simulink model "LUT_kidney_25"  (R2023b)
settings: Solver=FixedStepAuto  StartTime=0  StopTime=10.1  FixedStep=Timegap  RelTol=1e-3
model workspace (MAT data in the model file):
  T1_input = 1.34
(part 1 of 3)
settings Model: Creator=ppxmr2  LastModifiedBy=ppxmr2

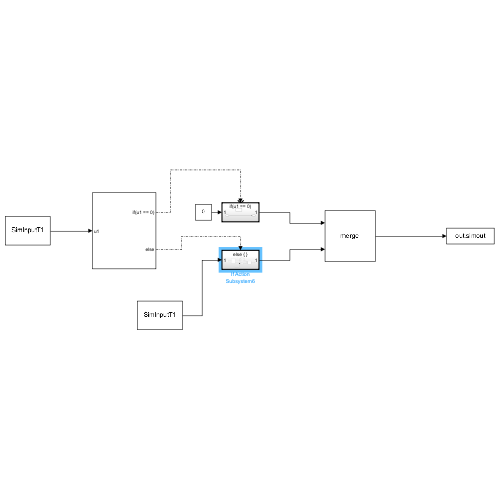
[thumbnail: Simulink's stored preview of the top-level diagram]
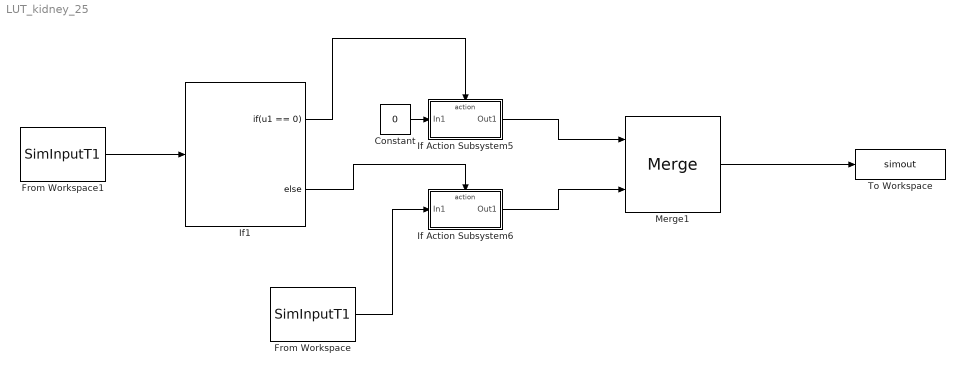
== system LUT_kidney_25 ==
  Constant : Constant  Value=0
  From Workspace : FromWorkspace  VariableName=SimInputT1  Interpolate=off  OutputAfterFinalValue=Setting to zero
  From Workspace1 : FromWorkspace  VariableName=SimInputT1  Interpolate=off  OutputAfterFinalValue=Setting to zero
  If Action Subsystem5 : Subsystem  TreatAsAtomicUnit=on
  If Action Subsystem6 : Subsystem  TreatAsAtomicUnit=on
  If1 : If  IfExpression=u1 == 0
  Merge1 : Merge
  To Workspace : ToWorkspace  VariableName=simout
  wires:
  From Workspace1/1 -> If1/1
  If1/1 -> If Action Subsystem5/Action
  If1/2 -> If Action Subsystem6/Action
  Constant/1 -> If Action Subsystem5/1(In1)
  If Action Subsystem5/1(Out1) -> Merge1/1
  If Action Subsystem6/1(Out1) -> Merge1/2
  Merge1/1 -> To Workspace/1
  From Workspace/1 -> If Action Subsystem6/1(In1)

== system LUT_kidney_25/If Action Subsystem5 ==
  In1 : Inport
  Action Port : ActionPort  ActionPortLabel=if(u1 == 0)
  Out1 : Outport
  wires:
  In1/1 -> Out1/1

== system LUT_kidney_25/If Action Subsystem6 ==
  In1 : Inport
  Action Port : ActionPort  ActionPortLabel=else
  From Workspace1 : FromWorkspace  VariableName=SimInputHR  Interpolate=off  OutputAfterFinalValue=Setting to zero
  If : If  IfExpression=u1 >= 1.495  ElseIfExpressions=u1 >= 0.995
  If Action Subsystem1 : Subsystem  TreatAsAtomicUnit=on
  If Action Subsystem2 : Subsystem  TreatAsAtomicUnit=on
  If Action Subsystem3 : Subsystem  TreatAsAtomicUnit=on
  Merge : Merge  Inputs=3
  Out1 : Outport
  wires:
  Merge/1 -> Out1/1
  From Workspace1/1 -> If/1
  If Action Subsystem1/1(Out1) -> Merge/2
  If Action Subsystem3/1(Out1) -> Merge/3
  In1/1 -> If Action Subsystem2/1(In1), If Action Subsystem1/1(In1), If Action Subsystem3/1(In1)
  If/1 -> If Action Subsystem2/Action
  If/2 -> If Action Subsystem1/Action
  If/3 -> If Action Subsystem3/Action
  If Action Subsystem2/1(Out1) -> Merge/1

== system LUT_kidney_25/If Action Subsystem6/If Action Subsystem1 ==
  In1 : Inport
  Action Port : ActionPort  ActionPortLabel=elseif(u1 >= 0.995)
  From Workspace2 : FromWorkspace  VariableName=SimInputHR  Interpolate=off  OutputAfterFinalValue=Setting to zero
  If Action Subsystem5 : Subsystem  TreatAsAtomicUnit=on
  If Action Subsystem6 : Subsystem  TreatAsAtomicUnit=on
  If Action Subsystem7 : Subsystem  TreatAsAtomicUnit=on
  If Action Subsystem8 : Subsystem  TreatAsAtomicUnit=on
  If Action Subsystem9 : Subsystem  TreatAsAtomicUnit=on
  If1 : If  IfExpression=u1 >= 1.395  ElseIfExpressions=u1 >= 1.295, u1 >= 1.195, u1 >= 1.095
  Merge1 : Merge  Inputs=5
  Out1 : Outport
  wires:
  In1/1 -> If Action Subsystem7/1(In2), If Action Subsystem8/1(In1), If Action Subsystem9/1(In1), If Action Subsystem5/1(In1), If Action Subsystem6/1(In1)
  From Workspace2/1 -> If1/1
  If Action Subsystem9/1(Out1) -> Merge1/1
  If Action Subsystem6/1(Out1) -> Merge1/5
  If Action Subsystem8/1(Out1) -> Merge1/2
  If Action Subsystem5/1(Out1) -> Merge1/4
  If1/4 -> If Action Subsystem5/Action
  If1/2 -> If Action Subsystem8/Action
  If1/3 -> If Action Subsystem7/Action
  If Action Subsystem7/1(Out2) -> Merge1/3
  If1/5 -> If Action Subsystem6/Action
  If1/1 -> If Action Subsystem9/Action
  Merge1/1 -> Out1/1

== system LUT_kidney_25/If Action Subsystem6/If Action Subsystem2 ==
  In1 : Inport
  Action Port : ActionPort  ActionPortLabel=if(u1 >= 1.495)
  From Workspace2 : FromWorkspace  VariableName=SimInputHR  Interpolate=off  OutputAfterFinalValue=Setting to zero
  If Action Subsystem5 : Subsystem  TreatAsAtomicUnit=on
  If Action Subsystem6 : Subsystem  TreatAsAtomicUnit=on
  If Action Subsystem7 : Subsystem  TreatAsAtomicUnit=on
  If Action Subsystem8 : Subsystem  TreatAsAtomicUnit=on
  If Action Subsystem9 : Subsystem  TreatAsAtomicUnit=on
  If1 : If  IfExpression=u1 >= 1.895  ElseIfExpressions=u1 >= 1.795, u1 >= 1.695, u1 >= 1.595
  Merge1 : Merge  Inputs=5
  Out1 : Outport
  wires:
  In1/1 -> If Action Subsystem9/1(In1), If Action Subsystem8/1(In1), If Action Subsystem7/1(In1), If Action Subsystem5/1(In1), If Action Subsystem6/1(In1)
  From Workspace2/1 -> If1/1
  If Action Subsystem9/1(Out1) -> Merge1/1
  If1/4 -> If Action Subsystem5/Action
  If1/2 -> If Action Subsystem8/Action
  If1/3 -> If Action Subsystem7/Action
  If1/5 -> If Action Subsystem6/Action
  If1/1 -> If Action Subsystem9/Action
  Merge1/1 -> Out1/1
  If Action Subsystem8/1(Out1) -> Merge1/2
  If Action Subsystem7/1(Out1) -> Merge1/3
  If Action Subsystem6/1(Out1) -> Merge1/5
  If Action Subsystem5/1(Out1) -> Merge1/4

== system LUT_kidney_25/If Action Subsystem6/If Action Subsystem3 ==
  In1 : Inport
  Action Port : ActionPort  ActionPortLabel=else
  From Workspace2 : FromWorkspace  VariableName=SimInputHR  Interpolate=off  OutputAfterFinalValue=Setting to zero
  If Action Subsystem5 : Subsystem  TreatAsAtomicUnit=on
  If Action Subsystem6 : Subsystem  TreatAsAtomicUnit=on
  If Action Subsystem7 : Subsystem  TreatAsAtomicUnit=on
  If Action Subsystem8 : Subsystem  TreatAsAtomicUnit=on
  If Action Subsystem9 : Subsystem  TreatAsAtomicUnit=on
  If1 : If  IfExpression=u1 >= 0.895  ElseIfExpressions=u1 >= 0.795, u1 >= 0.695, u1 >= 0595
  Merge1 : Merge  Inputs=5
  Out1 : Outport
  wires:
  In1/1 -> If Action Subsystem8/1(In1), If Action Subsystem9/1(In2), If Action Subsystem7/1(In1), If Action Subsystem5/1(In1), If Action Subsystem6/1(In1)
  From Workspace2/1 -> If1/1
  If Action Subsystem9/1(Out2) -> Merge1/1
  If Action Subsystem6/1(Out1) -> Merge1/5
  If Action Subsystem8/1(Out1) -> Merge1/2
  If Action Subsystem5/1(Out1) -> Merge1/4
  If1/4 -> If Action Subsystem5/Action
  If1/2 -> If Action Subsystem8/Action
  If1/3 -> If Action Subsystem7/Action
  If Action Subsystem7/1(Out1) -> Merge1/3
  If1/5 -> If Action Subsystem6/Action
  If1/1 -> If Action Subsystem9/Action
  Merge1/1 -> Out1/1

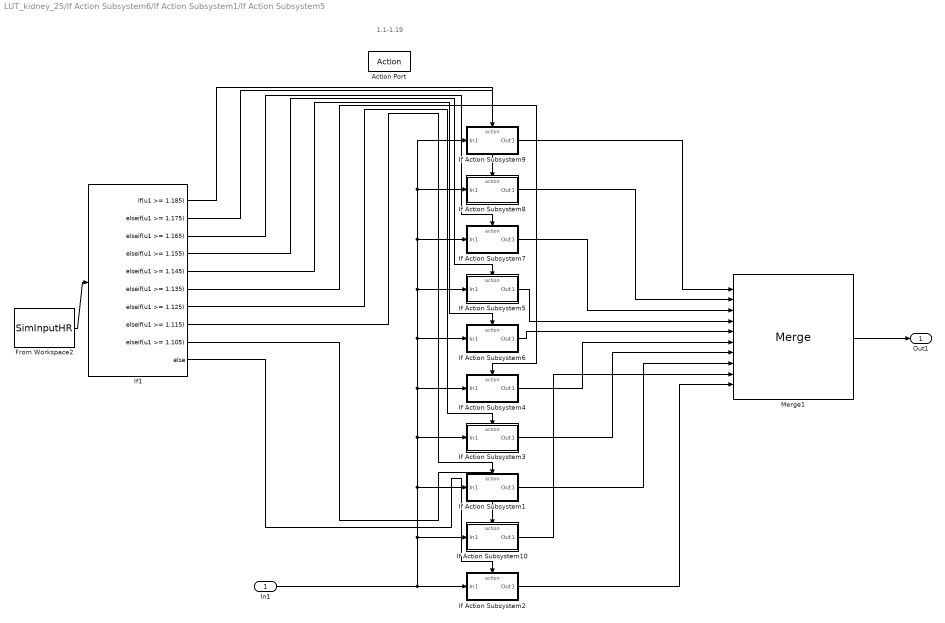
== system LUT_kidney_25/If Action Subsystem6/If Action Subsystem1/If Action Subsystem5 ==
  note: 1.1-1.19
  In1 : Inport
  Action Port : ActionPort  ActionPortLabel=elseif( u1 >= 1.095)
  From Workspace2 : FromWorkspace  VariableName=SimInputHR  Interpolate=off  OutputAfterFinalValue=Setting to zero
  If Action Subsystem1 : Subsystem  TreatAsAtomicUnit=on
  If Action Subsystem10 : Subsystem  TreatAsAtomicUnit=on
  If Action Subsystem2 : Subsystem  TreatAsAtomicUnit=on
  If Action Subsystem3 : Subsystem  TreatAsAtomicUnit=on
  If Action Subsystem4 : Subsystem  TreatAsAtomicUnit=on
  If Action Subsystem5 : Subsystem  TreatAsAtomicUnit=on
  If Action Subsystem6 : Subsystem  TreatAsAtomicUnit=on
  If Action Subsystem7 : Subsystem  TreatAsAtomicUnit=on
  If Action Subsystem8 : Subsystem  TreatAsAtomicUnit=on
  If Action Subsystem9 : Subsystem  TreatAsAtomicUnit=on
  If1 : If  IfExpression=u1 >= 1.185  ElseIfExpressions=u1 >= 1.175, u1 >= 1.165, u1 >= 1.155, u1 >= 1.145, u1 >= 1.135, u1 >= 1.125, u1 >= 1.115, u1 >= 1.105
  Merge1 : Merge  Inputs=10
  Out1 : Outport
  wires:
  If1/10 -> If Action Subsystem2/Action
  If Action Subsystem4/1(Out1) -> Merge1/6
  From Workspace2/1 -> If1/1
  If Action Subsystem6/1(Out1) -> Merge1/5
  Merge1/1 -> Out1/1
  If1/8 -> If Action Subsystem1/Action
  If Action Subsystem3/1(Out1) -> Merge1/7
  In1/1 -> If Action Subsystem1/1(In1), If Action Subsystem3/1(In1), If Action Subsystem4/1(In1), If Action Subsystem7/1(In1), If Action Subsystem8/1(In1), If Action Subsystem9/1(In1), If Action Subsystem5/1(In1), If Action Subsystem6/1(In1), If Action Subsystem10/1(In1), If Action Subsystem2/1(In1)
  If1/6 -> If Action Subsystem4/Action
  If Action Subsystem1/1(Out1) -> Merge1/8
  If1/4 -> If Action Subsystem5/Action
  If Action Subsystem8/1(Out1) -> Merge1/2
  If1/5 -> If Action Subsystem6/Action
  If Action Subsystem7/1(Out1) -> Merge1/3
  If1/3 -> If Action Subsystem7/Action
  If1/7 -> If Action Subsystem3/Action
  If Action Subsystem5/1(Out1) -> Merge1/4
  If Action Subsystem2/1(Out1) -> Merge1/10
  If1/2 -> If Action Subsystem8/Action
  If1/1 -> If Action Subsystem9/Action
  If Action Subsystem9/1(Out1) -> Merge1/1
  If1/9 -> If Action Subsystem10/Action
  If Action Subsystem10/1(Out1) -> Merge1/9

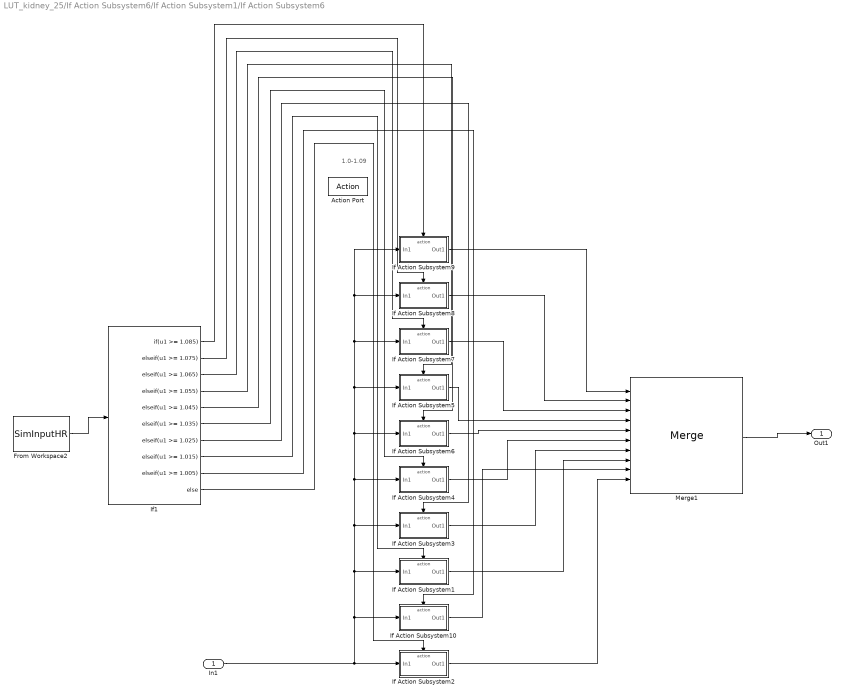
== system LUT_kidney_25/If Action Subsystem6/If Action Subsystem1/If Action Subsystem6 ==
  note: 1.0-1.09
  In1 : Inport
  Action Port : ActionPort  ActionPortLabel=else
  From Workspace2 : FromWorkspace  VariableName=SimInputHR  Interpolate=off  OutputAfterFinalValue=Setting to zero
  If Action Subsystem1 : Subsystem  TreatAsAtomicUnit=on
  If Action Subsystem10 : Subsystem  TreatAsAtomicUnit=on
  If Action Subsystem2 : Subsystem  TreatAsAtomicUnit=on
  If Action Subsystem3 : Subsystem  TreatAsAtomicUnit=on
  If Action Subsystem4 : Subsystem  TreatAsAtomicUnit=on
  If Action Subsystem5 : Subsystem  TreatAsAtomicUnit=on
  If Action Subsystem6 : Subsystem  TreatAsAtomicUnit=on
  If Action Subsystem7 : Subsystem  TreatAsAtomicUnit=on
  If Action Subsystem8 : Subsystem  TreatAsAtomicUnit=on
  If Action Subsystem9 : Subsystem  TreatAsAtomicUnit=on
  If1 : If  IfExpression=u1 >= 1.085  ElseIfExpressions=u1 >= 1.075, u1 >= 1.065, u1 >= 1.055, u1 >= 1.045, u1 >= 1.035, u1 >= 1.025, u1 >= 1.015, u1 >= 1.005
  Merge1 : Merge  Inputs=10
  Out1 : Outport
  wires:
  If1/10 -> If Action Subsystem2/Action
  If Action Subsystem4/1(Out1) -> Merge1/6
  From Workspace2/1 -> If1/1
  If Action Subsystem6/1(Out1) -> Merge1/5
  Merge1/1 -> Out1/1
  If1/8 -> If Action Subsystem1/Action
  If Action Subsystem3/1(Out1) -> Merge1/7
  In1/1 -> If Action Subsystem1/1(In1), If Action Subsystem3/1(In1), If Action Subsystem4/1(In1), If Action Subsystem7/1(In1), If Action Subsystem8/1(In1), If Action Subsystem9/1(In1), If Action Subsystem5/1(In1), If Action Subsystem6/1(In1), If Action Subsystem10/1(In1), If Action Subsystem2/1(In1)
  If1/6 -> If Action Subsystem4/Action
  If Action Subsystem1/1(Out1) -> Merge1/8
  If1/4 -> If Action Subsystem5/Action
  If Action Subsystem8/1(Out1) -> Merge1/2
  If1/5 -> If Action Subsystem6/Action
  If Action Subsystem7/1(Out1) -> Merge1/3
  If1/3 -> If Action Subsystem7/Action
  If1/7 -> If Action Subsystem3/Action
  If Action Subsystem5/1(Out1) -> Merge1/4
  If Action Subsystem2/1(Out1) -> Merge1/10
  If1/2 -> If Action Subsystem8/Action
  If1/1 -> If Action Subsystem9/Action
  If Action Subsystem9/1(Out1) -> Merge1/1
  If1/9 -> If Action Subsystem10/Action
  If Action Subsystem10/1(Out1) -> Merge1/9

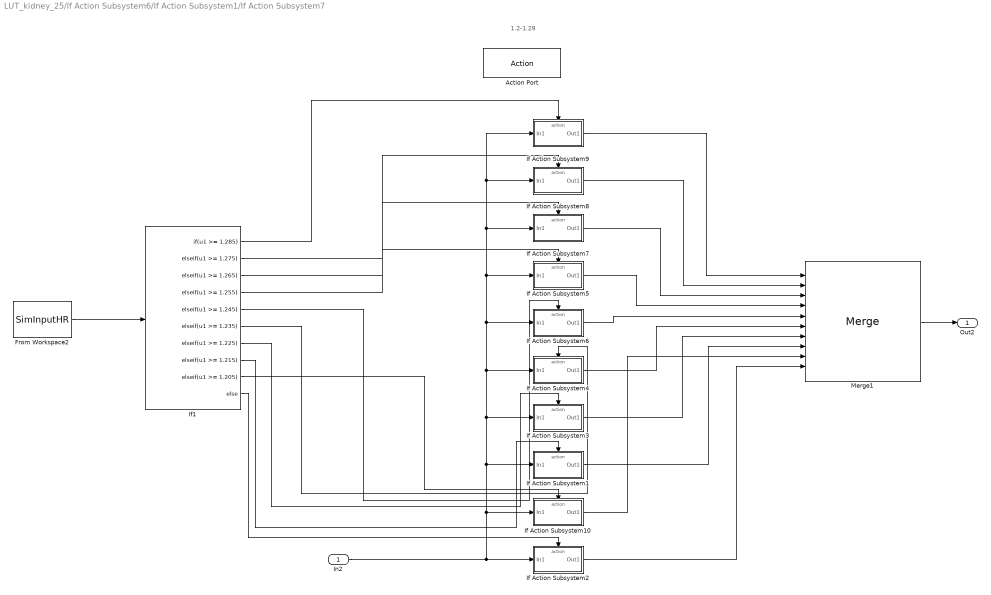
== system LUT_kidney_25/If Action Subsystem6/If Action Subsystem1/If Action Subsystem7 ==
  note: 1.2-1.29
  In2 : Inport
  Action Port : ActionPort  ActionPortLabel=elseif( u1 >= 1.195)
  From Workspace2 : FromWorkspace  VariableName=SimInputHR  Interpolate=off  OutputAfterFinalValue=Setting to zero
  If Action Subsystem1 : Subsystem  TreatAsAtomicUnit=on
  If Action Subsystem10 : Subsystem  TreatAsAtomicUnit=on
  If Action Subsystem2 : Subsystem  TreatAsAtomicUnit=on
  If Action Subsystem3 : Subsystem  TreatAsAtomicUnit=on
  If Action Subsystem4 : Subsystem  TreatAsAtomicUnit=on
  If Action Subsystem5 : Subsystem  TreatAsAtomicUnit=on
  If Action Subsystem6 : Subsystem  TreatAsAtomicUnit=on
  If Action Subsystem7 : Subsystem  TreatAsAtomicUnit=on
  If Action Subsystem8 : Subsystem  TreatAsAtomicUnit=on
  If Action Subsystem9 : Subsystem  TreatAsAtomicUnit=on
  If1 : If  IfExpression=u1 >= 1.285  ElseIfExpressions=u1 >= 1.275, u1 >= 1.265, u1 >= 1.255, u1 >= 1.245, u1 >= 1.235, u1 >= 1.225, u1 >= 1.215, u1 >= 1.205
  Merge1 : Merge  Inputs=10
  Out2 : Outport
  wires:
  If1/10 -> If Action Subsystem2/Action
  If Action Subsystem4/1(Out1) -> Merge1/6
  From Workspace2/1 -> If1/1
  If Action Subsystem6/1(Out1) -> Merge1/5
  Merge1/1 -> Out2/1
  If1/8 -> If Action Subsystem1/Action
  If Action Subsystem3/1(Out1) -> Merge1/7
  In2/1 -> If Action Subsystem1/1(In1), If Action Subsystem3/1(In1), If Action Subsystem4/1(In1), If Action Subsystem7/1(In1), If Action Subsystem8/1(In1), If Action Subsystem9/1(In1), If Action Subsystem5/1(In1), If Action Subsystem6/1(In1), If Action Subsystem10/1(In1), If Action Subsystem2/1(In1)
  If1/6 -> If Action Subsystem4/Action
  If Action Subsystem1/1(Out1) -> Merge1/8
  If1/4 -> If Action Subsystem5/Action
  If Action Subsystem8/1(Out1) -> Merge1/2
  If1/5 -> If Action Subsystem6/Action
  If Action Subsystem7/1(Out1) -> Merge1/3
  If1/3 -> If Action Subsystem7/Action
  If1/7 -> If Action Subsystem3/Action
  If Action Subsystem5/1(Out1) -> Merge1/4
  If Action Subsystem2/1(Out1) -> Merge1/10
  If1/2 -> If Action Subsystem8/Action
  If1/1 -> If Action Subsystem9/Action
  If Action Subsystem9/1(Out1) -> Merge1/1
  If Action Subsystem10/1(Out1) -> Merge1/9
  If1/9 -> If Action Subsystem10/Action

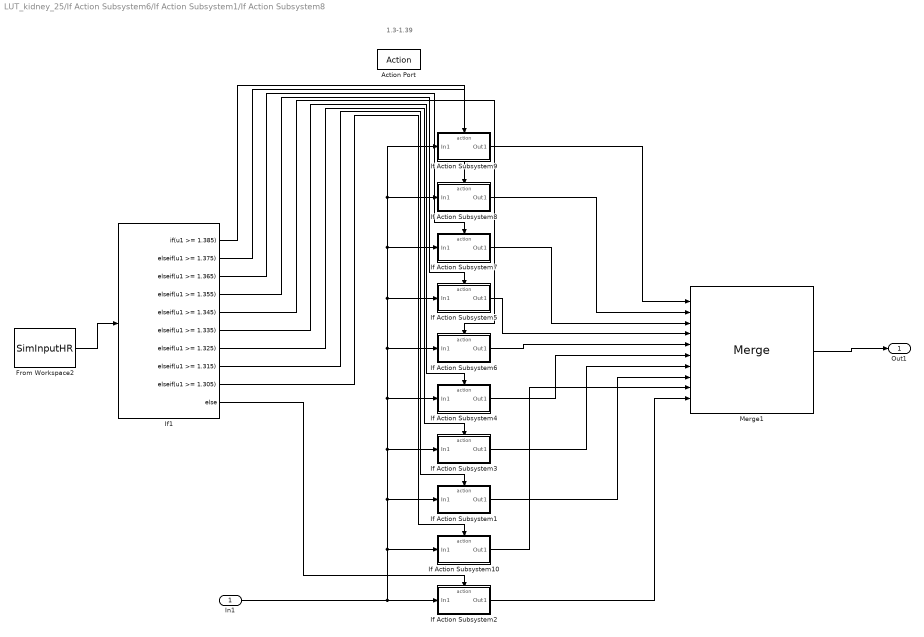
== system LUT_kidney_25/If Action Subsystem6/If Action Subsystem1/If Action Subsystem8 ==
  note: 1.3-1.39
  In1 : Inport
  Action Port : ActionPort  ActionPortLabel=elseif(u1 >= 1.295)
  From Workspace2 : FromWorkspace  VariableName=SimInputHR  Interpolate=off  OutputAfterFinalValue=Setting to zero
  If Action Subsystem1 : Subsystem  TreatAsAtomicUnit=on
  If Action Subsystem10 : Subsystem  TreatAsAtomicUnit=on
  If Action Subsystem2 : Subsystem  TreatAsAtomicUnit=on
  If Action Subsystem3 : Subsystem  TreatAsAtomicUnit=on
  If Action Subsystem4 : Subsystem  TreatAsAtomicUnit=on
  If Action Subsystem5 : Subsystem  TreatAsAtomicUnit=on
  If Action Subsystem6 : Subsystem  TreatAsAtomicUnit=on
  If Action Subsystem7 : Subsystem  TreatAsAtomicUnit=on
  If Action Subsystem8 : Subsystem  TreatAsAtomicUnit=on
  If Action Subsystem9 : Subsystem  TreatAsAtomicUnit=on
  If1 : If  IfExpression=u1 >= 1.385  ElseIfExpressions=u1 >= 1.375, u1 >= 1.365, u1 >= 1.355, u1 >= 1.345, u1 >= 1.335, u1 >= 1.325, u1 >= 1.315, u1 >= 1.305
  Merge1 : Merge  Inputs=10
  Out1 : Outport
  wires:
  If1/10 -> If Action Subsystem2/Action
  If Action Subsystem4/1(Out1) -> Merge1/6
  From Workspace2/1 -> If1/1
  If Action Subsystem6/1(Out1) -> Merge1/5
  Merge1/1 -> Out1/1
  If1/8 -> If Action Subsystem1/Action
  If Action Subsystem3/1(Out1) -> Merge1/7
  In1/1 -> If Action Subsystem1/1(In1), If Action Subsystem3/1(In1), If Action Subsystem4/1(In1), If Action Subsystem7/1(In1), If Action Subsystem8/1(In1), If Action Subsystem9/1(In1), If Action Subsystem5/1(In1), If Action Subsystem6/1(In1), If Action Subsystem10/1(In1), If Action Subsystem2/1(In1)
  If1/6 -> If Action Subsystem4/Action
  If Action Subsystem1/1(Out1) -> Merge1/8
  If1/4 -> If Action Subsystem5/Action
  If Action Subsystem8/1(Out1) -> Merge1/2
  If1/5 -> If Action Subsystem6/Action
  If Action Subsystem7/1(Out1) -> Merge1/3
  If1/3 -> If Action Subsystem7/Action
  If1/7 -> If Action Subsystem3/Action
  If Action Subsystem5/1(Out1) -> Merge1/4
  If Action Subsystem2/1(Out1) -> Merge1/10
  If1/2 -> If Action Subsystem8/Action
  If1/1 -> If Action Subsystem9/Action
  If Action Subsystem9/1(Out1) -> Merge1/1
  If1/9 -> If Action Subsystem10/Action
  If Action Subsystem10/1(Out1) -> Merge1/9

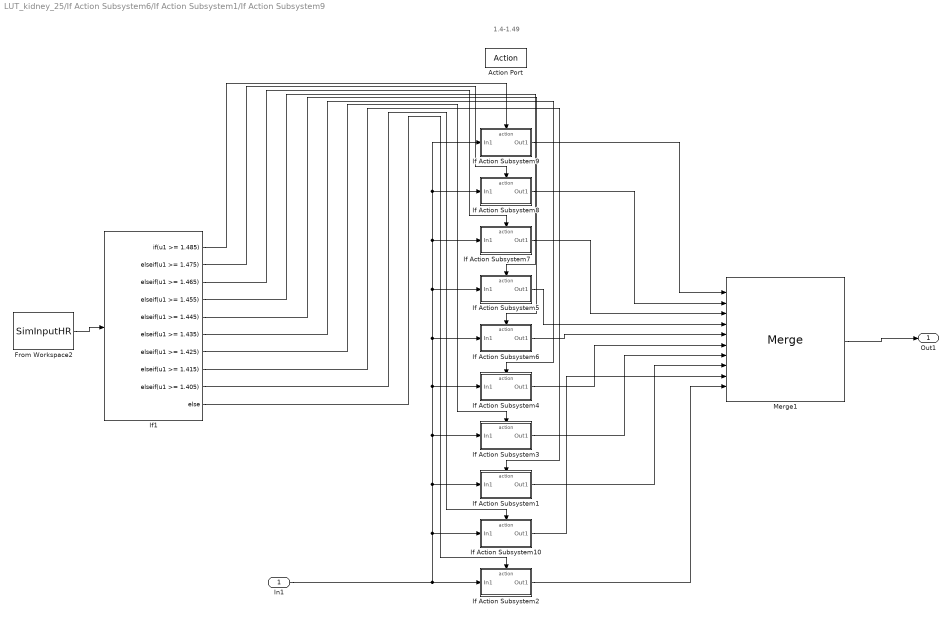
== system LUT_kidney_25/If Action Subsystem6/If Action Subsystem1/If Action Subsystem9 ==
  note: 1.4-1.49
  In1 : Inport
  Action Port : ActionPort  ActionPortLabel=if(u1 >= 1.395)
  From Workspace2 : FromWorkspace  VariableName=SimInputHR  Interpolate=off  OutputAfterFinalValue=Setting to zero
  If Action Subsystem1 : Subsystem  TreatAsAtomicUnit=on
  If Action Subsystem10 : Subsystem  TreatAsAtomicUnit=on
  If Action Subsystem2 : Subsystem  TreatAsAtomicUnit=on
  If Action Subsystem3 : Subsystem  TreatAsAtomicUnit=on
  If Action Subsystem4 : Subsystem  TreatAsAtomicUnit=on
  If Action Subsystem5 : Subsystem  TreatAsAtomicUnit=on
  If Action Subsystem6 : Subsystem  TreatAsAtomicUnit=on
  If Action Subsystem7 : Subsystem  TreatAsAtomicUnit=on
  If Action Subsystem8 : Subsystem  TreatAsAtomicUnit=on
  If Action Subsystem9 : Subsystem  TreatAsAtomicUnit=on
  If1 : If  IfExpression=u1 >= 1.485  ElseIfExpressions=u1 >= 1.475, u1 >= 1.465, u1 >= 1.455, u1 >= 1.445, u1 >= 1.435, u1 >= 1.425, u1 >= 1.415, u1 >= 1.405
  Merge1 : Merge  Inputs=10
  Out1 : Outport
  wires:
  If1/10 -> If Action Subsystem2/Action
  If Action Subsystem4/1(Out1) -> Merge1/6
  From Workspace2/1 -> If1/1
  If Action Subsystem6/1(Out1) -> Merge1/5
  Merge1/1 -> Out1/1
  If1/8 -> If Action Subsystem1/Action
  If Action Subsystem3/1(Out1) -> Merge1/7
  In1/1 -> If Action Subsystem10/1(In1), If Action Subsystem1/1(In1), If Action Subsystem3/1(In1), If Action Subsystem4/1(In1), If Action Subsystem7/1(In1), If Action Subsystem8/1(In1), If Action Subsystem9/1(In1), If Action Subsystem5/1(In1), If Action Subsystem6/1(In1), If Action Subsystem2/1(In1)
  If1/6 -> If Action Subsystem4/Action
  If Action Subsystem1/1(Out1) -> Merge1/8
  If1/4 -> If Action Subsystem5/Action
  If Action Subsystem8/1(Out1) -> Merge1/2
  If1/5 -> If Action Subsystem6/Action
  If Action Subsystem7/1(Out1) -> Merge1/3
  If1/3 -> If Action Subsystem7/Action
  If1/7 -> If Action Subsystem3/Action
  If Action Subsystem5/1(Out1) -> Merge1/4
  If Action Subsystem2/1(Out1) -> Merge1/10
  If1/2 -> If Action Subsystem8/Action
  If1/1 -> If Action Subsystem9/Action
  If Action Subsystem9/1(Out1) -> Merge1/1
  If1/9 -> If Action Subsystem10/Action
  If Action Subsystem10/1(Out1) -> Merge1/9

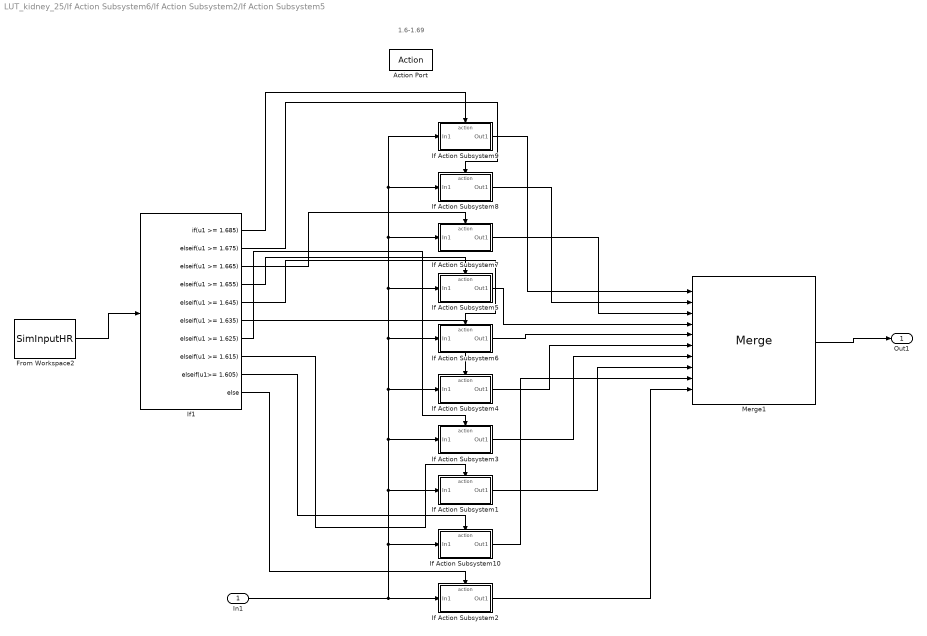
== system LUT_kidney_25/If Action Subsystem6/If Action Subsystem2/If Action Subsystem5 ==
  note: 1.6-1.69
  In1 : Inport
  Action Port : ActionPort  ActionPortLabel=elseif( u1 >= 1.595)
  From Workspace2 : FromWorkspace  VariableName=SimInputHR  Interpolate=off  OutputAfterFinalValue=Setting to zero
  If Action Subsystem1 : Subsystem  TreatAsAtomicUnit=on
  If Action Subsystem10 : Subsystem  TreatAsAtomicUnit=on
  If Action Subsystem2 : Subsystem  TreatAsAtomicUnit=on
  If Action Subsystem3 : Subsystem  TreatAsAtomicUnit=on
  If Action Subsystem4 : Subsystem  TreatAsAtomicUnit=on
  If Action Subsystem5 : Subsystem  TreatAsAtomicUnit=on
  If Action Subsystem6 : Subsystem  TreatAsAtomicUnit=on
  If Action Subsystem7 : Subsystem  TreatAsAtomicUnit=on
  If Action Subsystem8 : Subsystem  TreatAsAtomicUnit=on
  If Action Subsystem9 : Subsystem  TreatAsAtomicUnit=on
  If1 : If  IfExpression=u1 >= 1.685  ElseIfExpressions=u1 >= 1.675, u1 >= 1.665, u1 >= 1.655, u1 >= 1.645, u1 >= 1.635, u1 >= 1.625, u1 >= 1.615, u1>= 1.605
  Merge1 : Merge  Inputs=10
  Out1 : Outport
  wires:
  If1/2 -> If Action Subsystem8/Action
  If Action Subsystem5/1(Out1) -> Merge1/4
  If1/3 -> If Action Subsystem7/Action
  If Action Subsystem9/1(Out1) -> Merge1/1
  If1/7 -> If Action Subsystem3/Action
  If1/5 -> If Action Subsystem6/Action
  If1/1 -> If Action Subsystem9/Action
  If Action Subsystem4/1(Out1) -> Merge1/6
  If1/10 -> If Action Subsystem2/Action
  If Action Subsystem8/1(Out1) -> Merge1/2
  If1/4 -> If Action Subsystem5/Action
  In1/1 -> If Action Subsystem10/1(In1), If Action Subsystem1/1(In1), If Action Subsystem3/1(In1), If Action Subsystem4/1(In1), If Action Subsystem7/1(In1), If Action Subsystem8/1(In1), If Action Subsystem9/1(In1), If Action Subsystem5/1(In1), If Action Subsystem6/1(In1), If Action Subsystem2/1(In1)
  If Action Subsystem1/1(Out1) -> Merge1/8
  If Action Subsystem2/1(Out1) -> Merge1/10
  If1/8 -> If Action Subsystem1/Action
  If Action Subsystem3/1(Out1) -> Merge1/7
  If1/6 -> If Action Subsystem4/Action
  From Workspace2/1 -> If1/1
  Merge1/1 -> Out1/1
  If Action Subsystem6/1(Out1) -> Merge1/5
  If Action Subsystem7/1(Out1) -> Merge1/3
  If1/9 -> If Action Subsystem10/Action
  If Action Subsystem10/1(Out1) -> Merge1/9

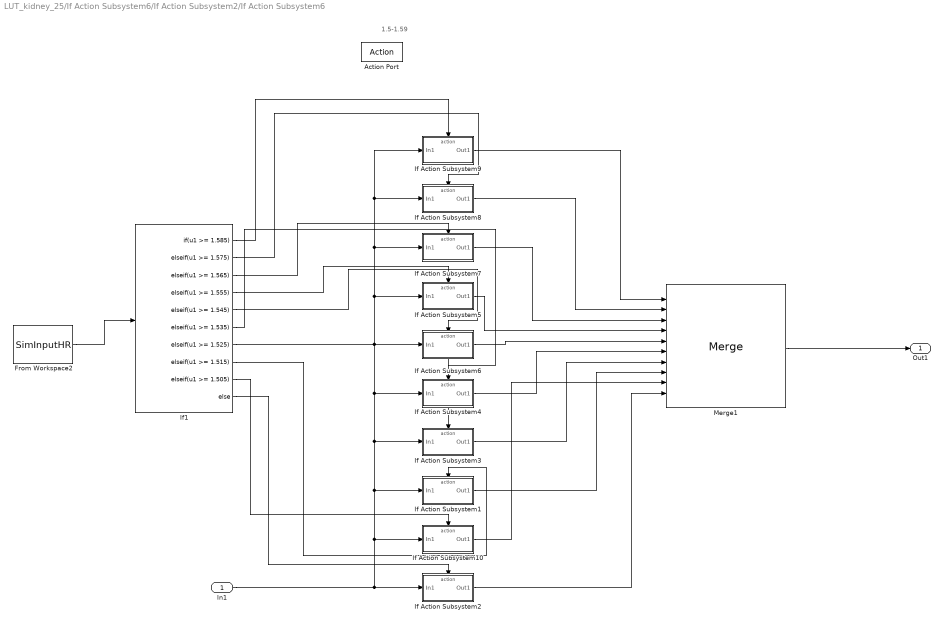
== system LUT_kidney_25/If Action Subsystem6/If Action Subsystem2/If Action Subsystem6 ==
  note: 1.5-1.59
  In1 : Inport
  Action Port : ActionPort  ActionPortLabel=else
  From Workspace2 : FromWorkspace  VariableName=SimInputHR  Interpolate=off  OutputAfterFinalValue=Setting to zero
  If Action Subsystem1 : Subsystem  TreatAsAtomicUnit=on
  If Action Subsystem10 : Subsystem  TreatAsAtomicUnit=on
  If Action Subsystem2 : Subsystem  TreatAsAtomicUnit=on
  If Action Subsystem3 : Subsystem  TreatAsAtomicUnit=on
  If Action Subsystem4 : Subsystem  TreatAsAtomicUnit=on
  If Action Subsystem5 : Subsystem  TreatAsAtomicUnit=on
  If Action Subsystem6 : Subsystem  TreatAsAtomicUnit=on
  If Action Subsystem7 : Subsystem  TreatAsAtomicUnit=on
  If Action Subsystem8 : Subsystem  TreatAsAtomicUnit=on
  If Action Subsystem9 : Subsystem  TreatAsAtomicUnit=on
  If1 : If  IfExpression=u1 >= 1.585  ElseIfExpressions=u1 >= 1.575, u1 >= 1.565, u1 >= 1.555, u1 >= 1.545, u1 >= 1.535, u1 >= 1.525, u1 >= 1.515, u1 >= 1.505
  Merge1 : Merge  Inputs=10
  Out1 : Outport
  wires:
  If1/2 -> If Action Subsystem8/Action
  If Action Subsystem5/1(Out1) -> Merge1/4
  If1/3 -> If Action Subsystem7/Action
  If Action Subsystem9/1(Out1) -> Merge1/1
  If1/7 -> If Action Subsystem3/Action
  If1/5 -> If Action Subsystem6/Action
  If1/1 -> If Action Subsystem9/Action
  If Action Subsystem4/1(Out1) -> Merge1/6
  If1/10 -> If Action Subsystem2/Action
  If Action Subsystem8/1(Out1) -> Merge1/2
  If1/4 -> If Action Subsystem5/Action
  In1/1 -> If Action Subsystem10/1(In1), If Action Subsystem1/1(In1), If Action Subsystem3/1(In1), If Action Subsystem4/1(In1), If Action Subsystem7/1(In1), If Action Subsystem8/1(In1), If Action Subsystem9/1(In1), If Action Subsystem5/1(In1), If Action Subsystem6/1(In1), If Action Subsystem2/1(In1)
  If Action Subsystem1/1(Out1) -> Merge1/8
  If Action Subsystem2/1(Out1) -> Merge1/10
  If1/8 -> If Action Subsystem1/Action
  If Action Subsystem3/1(Out1) -> Merge1/7
  If1/6 -> If Action Subsystem4/Action
  From Workspace2/1 -> If1/1
  Merge1/1 -> Out1/1
  If Action Subsystem6/1(Out1) -> Merge1/5
  If Action Subsystem7/1(Out1) -> Merge1/3
  If1/9 -> If Action Subsystem10/Action
  If Action Subsystem10/1(Out1) -> Merge1/9

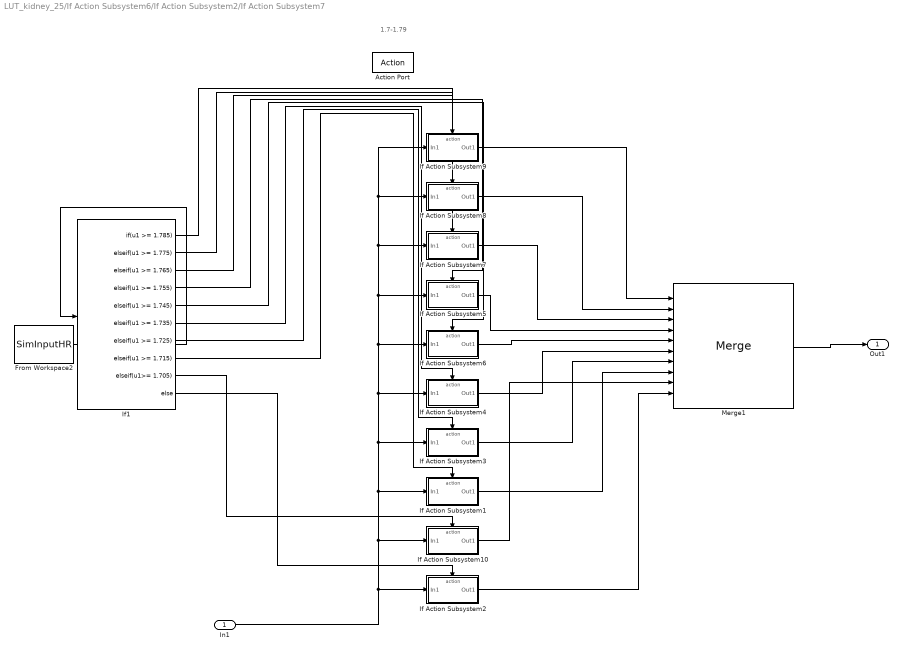
== system LUT_kidney_25/If Action Subsystem6/If Action Subsystem2/If Action Subsystem7 ==
  note: 1.7-1.79
  In1 : Inport
  Action Port : ActionPort  ActionPortLabel=elseif( u1 >= 1.695)
  From Workspace2 : FromWorkspace  VariableName=SimInputHR  Interpolate=off  OutputAfterFinalValue=Setting to zero
  If Action Subsystem1 : Subsystem  TreatAsAtomicUnit=on
  If Action Subsystem10 : Subsystem  TreatAsAtomicUnit=on
  If Action Subsystem2 : Subsystem  TreatAsAtomicUnit=on
  If Action Subsystem3 : Subsystem  TreatAsAtomicUnit=on
  If Action Subsystem4 : Subsystem  TreatAsAtomicUnit=on
  If Action Subsystem5 : Subsystem  TreatAsAtomicUnit=on
  If Action Subsystem6 : Subsystem  TreatAsAtomicUnit=on
  If Action Subsystem7 : Subsystem  TreatAsAtomicUnit=on
  If Action Subsystem8 : Subsystem  TreatAsAtomicUnit=on
  If Action Subsystem9 : Subsystem  TreatAsAtomicUnit=on
  If1 : If  IfExpression=u1 >= 1.785  ElseIfExpressions=u1 >= 1.775, u1 >= 1.765, u1 >= 1.755, u1 >= 1.745, u1 >= 1.735, u1 >= 1.725, u1 >= 1.715, u1>= 1.705
  Merge1 : Merge  Inputs=10
  Out1 : Outport
  wires:
  If1/2 -> If Action Subsystem8/Action
  If Action Subsystem5/1(Out1) -> Merge1/4
  If1/3 -> If Action Subsystem7/Action
  If Action Subsystem9/1(Out1) -> Merge1/1
  If1/7 -> If Action Subsystem3/Action
  If1/5 -> If Action Subsystem6/Action
  If1/1 -> If Action Subsystem9/Action
  If Action Subsystem4/1(Out1) -> Merge1/6
  If1/10 -> If Action Subsystem2/Action
  If Action Subsystem8/1(Out1) -> Merge1/2
  If1/4 -> If Action Subsystem5/Action
  In1/1 -> If Action Subsystem10/1(In1), If Action Subsystem1/1(In1), If Action Subsystem3/1(In1), If Action Subsystem4/1(In1), If Action Subsystem7/1(In1), If Action Subsystem8/1(In1), If Action Subsystem9/1(In1), If Action Subsystem5/1(In1), If Action Subsystem6/1(In1), If Action Subsystem2/1(In1)
  If Action Subsystem1/1(Out1) -> Merge1/8
  If Action Subsystem2/1(Out1) -> Merge1/10
  If1/8 -> If Action Subsystem1/Action
  If Action Subsystem3/1(Out1) -> Merge1/7
  If1/6 -> If Action Subsystem4/Action
  From Workspace2/1 -> If1/1
  Merge1/1 -> Out1/1
  If Action Subsystem6/1(Out1) -> Merge1/5
  If Action Subsystem7/1(Out1) -> Merge1/3
  If Action Subsystem10/1(Out1) -> Merge1/9
  If1/9 -> If Action Subsystem10/Action

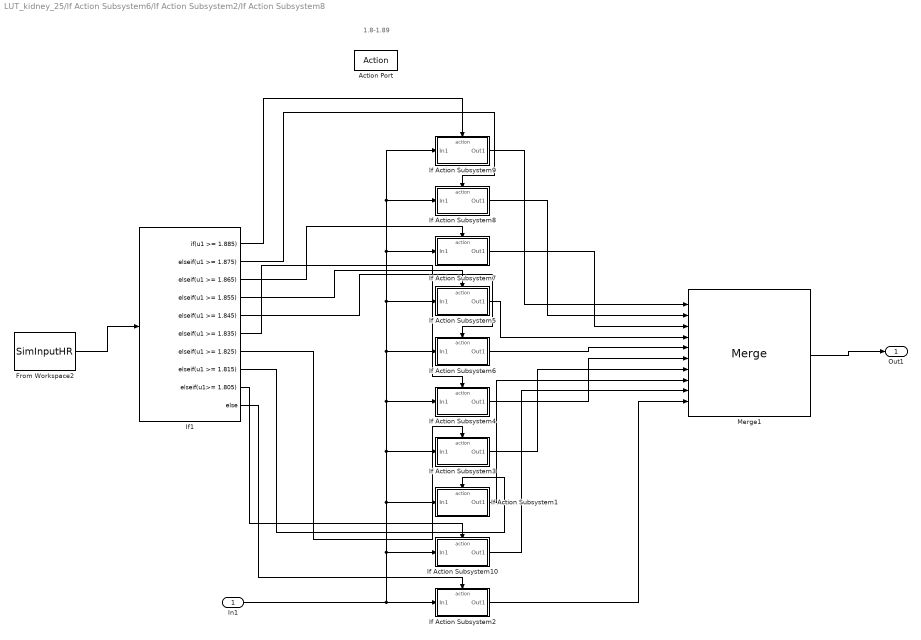
== system LUT_kidney_25/If Action Subsystem6/If Action Subsystem2/If Action Subsystem8 ==
  note: 1.8-1.89
  In1 : Inport
  Action Port : ActionPort  ActionPortLabel=elseif(u1 >= 1.795)
  From Workspace2 : FromWorkspace  VariableName=SimInputHR  Interpolate=off  OutputAfterFinalValue=Setting to zero
  If Action Subsystem1 : Subsystem  TreatAsAtomicUnit=on
  If Action Subsystem10 : Subsystem  TreatAsAtomicUnit=on
  If Action Subsystem2 : Subsystem  TreatAsAtomicUnit=on
  If Action Subsystem3 : Subsystem  TreatAsAtomicUnit=on
  If Action Subsystem4 : Subsystem  TreatAsAtomicUnit=on
  If Action Subsystem5 : Subsystem  TreatAsAtomicUnit=on
  If Action Subsystem6 : Subsystem  TreatAsAtomicUnit=on
  If Action Subsystem7 : Subsystem  TreatAsAtomicUnit=on
  If Action Subsystem8 : Subsystem  TreatAsAtomicUnit=on
  If Action Subsystem9 : Subsystem  TreatAsAtomicUnit=on
  If1 : If  IfExpression=u1 >= 1.885  ElseIfExpressions=u1 >= 1.875, u1 >= 1.865, u1 >= 1.855, u1 >= 1.845, u1 >= 1.835, u1 >= 1.825, u1 >= 1.815, u1>= 1.805
  Merge1 : Merge  Inputs=10
  Out1 : Outport
  wires:
  If1/2 -> If Action Subsystem8/Action
  If Action Subsystem5/1(Out1) -> Merge1/4
  If1/3 -> If Action Subsystem7/Action
  If Action Subsystem9/1(Out1) -> Merge1/1
  If1/7 -> If Action Subsystem3/Action
  If1/5 -> If Action Subsystem6/Action
  If1/1 -> If Action Subsystem9/Action
  If Action Subsystem4/1(Out1) -> Merge1/6
  If1/10 -> If Action Subsystem2/Action
  If Action Subsystem8/1(Out1) -> Merge1/2
  If1/4 -> If Action Subsystem5/Action
  In1/1 -> If Action Subsystem10/1(In1), If Action Subsystem1/1(In1), If Action Subsystem3/1(In1), If Action Subsystem4/1(In1), If Action Subsystem7/1(In1), If Action Subsystem8/1(In1), If Action Subsystem9/1(In1), If Action Subsystem5/1(In1), If Action Subsystem6/1(In1), If Action Subsystem2/1(In1)
  If Action Subsystem1/1(Out1) -> Merge1/8
  If Action Subsystem2/1(Out1) -> Merge1/10
  If1/8 -> If Action Subsystem1/Action
  If Action Subsystem3/1(Out1) -> Merge1/7
  If1/6 -> If Action Subsystem4/Action
  From Workspace2/1 -> If1/1
  Merge1/1 -> Out1/1
  If Action Subsystem6/1(Out1) -> Merge1/5
  If Action Subsystem7/1(Out1) -> Merge1/3
  If1/9 -> If Action Subsystem10/Action
  If Action Subsystem10/1(Out1) -> Merge1/9

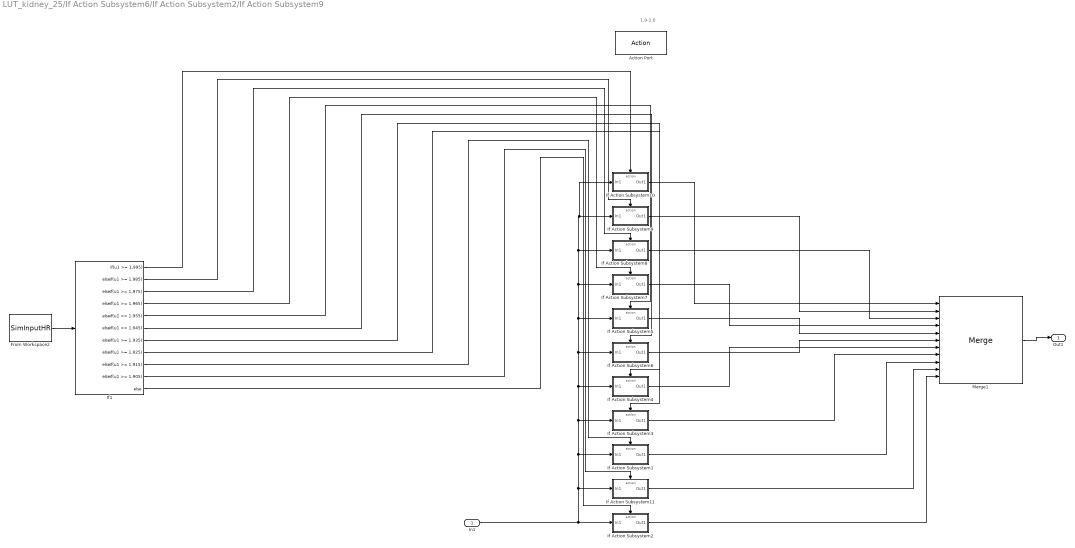
== system LUT_kidney_25/If Action Subsystem6/If Action Subsystem2/If Action Subsystem9 ==
  note: 1.9-2.0
  In1 : Inport
  Action Port : ActionPort  ActionPortLabel=if(u1 >= 1.895)
  From Workspace2 : FromWorkspace  VariableName=SimInputHR  Interpolate=off  OutputAfterFinalValue=Setting to zero
  If Action Subsystem1 : Subsystem  TreatAsAtomicUnit=on
  If Action Subsystem10 : Subsystem  TreatAsAtomicUnit=on
  If Action Subsystem11 : Subsystem  TreatAsAtomicUnit=on
  If Action Subsystem2 : Subsystem  TreatAsAtomicUnit=on
  If Action Subsystem3 : Subsystem  TreatAsAtomicUnit=on
  If Action Subsystem4 : Subsystem  TreatAsAtomicUnit=on
  If Action Subsystem5 : Subsystem  TreatAsAtomicUnit=on
  If Action Subsystem6 : Subsystem  TreatAsAtomicUnit=on
  If Action Subsystem7 : Subsystem  TreatAsAtomicUnit=on
  If Action Subsystem8 : Subsystem  TreatAsAtomicUnit=on
  If Action Subsystem9 : Subsystem  TreatAsAtomicUnit=on
  If1 : If  IfExpression=u1 >= 1.995  ElseIfExpressions=u1 >= 1.985, u1 >= 1.975, u1 >= 1.965, u1 >= 1.955, u1 >= 1.945, u1 >= 1.935, u1 >= 1.925, u1 >= 1.915, u1 >= 1.905
  Merge1 : Merge  Inputs=11
  Out1 : Outport
  wires:
  Merge1/1 -> Out1/1
  From Workspace2/1 -> If1/1
  If1/2 -> If Action Subsystem9/Action
  If1/3 -> If Action Subsystem8/Action
  If1/4 -> If Action Subsystem7/Action
  If1/5 -> If Action Subsystem5/Action
  If1/6 -> If Action Subsystem6/Action
  If1/7 -> If Action Subsystem4/Action
  If1/8 -> If Action Subsystem3/Action
  If1/9 -> If Action Subsystem1/Action
  If1/11 -> If Action Subsystem2/Action
  If Action Subsystem9/1(Out1) -> Merge1/2
  If Action Subsystem8/1(Out1) -> Merge1/3
  If Action Subsystem7/1(Out1) -> Merge1/4
  If Action Subsystem5/1(Out1) -> Merge1/5
  If Action Subsystem6/1(Out1) -> Merge1/6
  If Action Subsystem4/1(Out1) -> Merge1/7
  If Action Subsystem3/1(Out1) -> Merge1/8
  If Action Subsystem2/1(Out1) -> Merge1/11
  If Action Subsystem1/1(Out1) -> Merge1/9
  In1/1 -> If Action Subsystem1/1(In1), If Action Subsystem3/1(In1), If Action Subsystem4/1(In1), If Action Subsystem7/1(In1), If Action Subsystem8/1(In1), If Action Subsystem10/1(In1), If Action Subsystem9/1(In1), If Action Subsystem5/1(In1), If Action Subsystem6/1(In1), If Action Subsystem11/1(In1), If Action Subsystem2/1(In1)
  If1/1 -> If Action Subsystem10/Action
  If Action Subsystem10/1(Out1) -> Merge1/1
  If1/10 -> If Action Subsystem11/Action
  If Action Subsystem11/1(Out1) -> Merge1/10

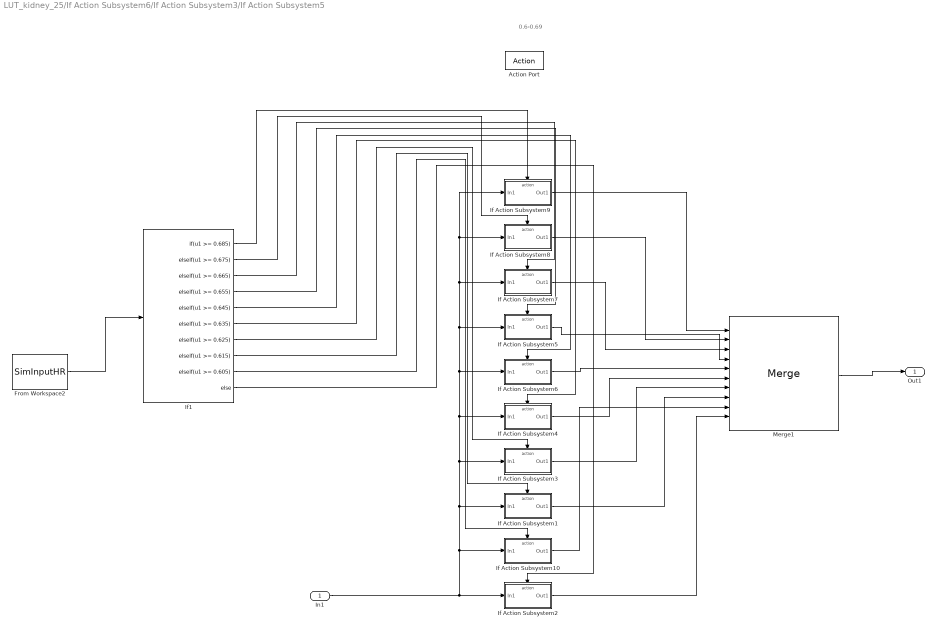
== system LUT_kidney_25/If Action Subsystem6/If Action Subsystem3/If Action Subsystem5 ==
  note: 0.6-0.69
  In1 : Inport
  Action Port : ActionPort  ActionPortLabel=elseif( u1 >= 0595)
  From Workspace2 : FromWorkspace  VariableName=SimInputHR  Interpolate=off  OutputAfterFinalValue=Setting to zero
  If Action Subsystem1 : Subsystem  TreatAsAtomicUnit=on
  If Action Subsystem10 : Subsystem  TreatAsAtomicUnit=on
  If Action Subsystem2 : Subsystem  TreatAsAtomicUnit=on
  If Action Subsystem3 : Subsystem  TreatAsAtomicUnit=on
  If Action Subsystem4 : Subsystem  TreatAsAtomicUnit=on
  If Action Subsystem5 : Subsystem  TreatAsAtomicUnit=on
  If Action Subsystem6 : Subsystem  TreatAsAtomicUnit=on
  If Action Subsystem7 : Subsystem  TreatAsAtomicUnit=on
  If Action Subsystem8 : Subsystem  TreatAsAtomicUnit=on
  If Action Subsystem9 : Subsystem  TreatAsAtomicUnit=on
  If1 : If  IfExpression=u1 >= 0.685  ElseIfExpressions=u1 >= 0.675, u1 >= 0.665, u1 >= 0.655, u1 >= 0.645, u1 >= 0.635, u1 >= 0.625, u1 >= 0.615, u1 >= 0.605
  Merge1 : Merge  Inputs=10
  Out1 : Outport
  wires:
  If1/10 -> If Action Subsystem2/Action
  If Action Subsystem4/1(Out1) -> Merge1/6
  From Workspace2/1 -> If1/1
  If Action Subsystem6/1(Out1) -> Merge1/5
  Merge1/1 -> Out1/1
  If1/8 -> If Action Subsystem1/Action
  If Action Subsystem3/1(Out1) -> Merge1/7
  In1/1 -> If Action Subsystem1/1(In1), If Action Subsystem3/1(In1), If Action Subsystem4/1(In1), If Action Subsystem7/1(In1), If Action Subsystem8/1(In1), If Action Subsystem9/1(In1), If Action Subsystem5/1(In1), If Action Subsystem6/1(In1), If Action Subsystem10/1(In1), If Action Subsystem2/1(In1)
  If1/6 -> If Action Subsystem4/Action
  If Action Subsystem1/1(Out1) -> Merge1/8
  If1/4 -> If Action Subsystem5/Action
  If Action Subsystem8/1(Out1) -> Merge1/2
  If1/5 -> If Action Subsystem6/Action
  If Action Subsystem7/1(Out1) -> Merge1/3
  If1/3 -> If Action Subsystem7/Action
  If1/7 -> If Action Subsystem3/Action
  If Action Subsystem5/1(Out1) -> Merge1/4
  If Action Subsystem2/1(Out1) -> Merge1/10
  If1/2 -> If Action Subsystem8/Action
  If1/1 -> If Action Subsystem9/Action
  If Action Subsystem9/1(Out1) -> Merge1/1
  If Action Subsystem10/1(Out1) -> Merge1/9
  If1/9 -> If Action Subsystem10/Action

== system LUT_kidney_25/If Action Subsystem6/If Action Subsystem3/If Action Subsystem6 ==
  note: 0.5-0.59
  In1 : Inport
  Action Port : ActionPort  ActionPortLabel=else
  From Workspace2 : FromWorkspace  VariableName=SimInputHR  Interpolate=off  OutputAfterFinalValue=Setting to zero
  If Action Subsystem1 : Subsystem  TreatAsAtomicUnit=on
  If Action Subsystem10 : Subsystem  TreatAsAtomicUnit=on
  If Action Subsystem2 : Subsystem  TreatAsAtomicUnit=on
  If Action Subsystem3 : Subsystem  TreatAsAtomicUnit=on
  If Action Subsystem4 : Subsystem  TreatAsAtomicUnit=on
  If Action Subsystem5 : Subsystem  TreatAsAtomicUnit=on
  If Action Subsystem6 : Subsystem  TreatAsAtomicUnit=on
  If Action Subsystem7 : Subsystem  TreatAsAtomicUnit=on
  If Action Subsystem8 : Subsystem  TreatAsAtomicUnit=on
  If Action Subsystem9 : Subsystem  TreatAsAtomicUnit=on
  If1 : If  IfExpression=u1 >= 0.585  ElseIfExpressions=u1 >= 0.575, u1 >= 0.565, u1 >= 0.555, u1 >= 0.545, u1 >= 0.535, u1 >= 0.525, u1 >= 0.515, u1 >= 0.505
  Merge1 : Merge  Inputs=10
  Out1 : Outport
  wires:
  If1/10 -> If Action Subsystem2/Action
  If Action Subsystem4/1(Out1) -> Merge1/6
  From Workspace2/1 -> If1/1
  If Action Subsystem6/1(Out1) -> Merge1/5
  Merge1/1 -> Out1/1
  If1/8 -> If Action Subsystem1/Action
  If Action Subsystem3/1(Out1) -> Merge1/7
  In1/1 -> If Action Subsystem1/1(In1), If Action Subsystem3/1(In1), If Action Subsystem4/1(In1), If Action Subsystem7/1(In1), If Action Subsystem8/1(In1), If Action Subsystem9/1(In1), If Action Subsystem5/1(In1), If Action Subsystem6/1(In1), If Action Subsystem10/1(In1), If Action Subsystem2/1(In1)
  If1/6 -> If Action Subsystem4/Action
  If Action Subsystem1/1(Out1) -> Merge1/8
  If1/4 -> If Action Subsystem5/Action
  If Action Subsystem8/1(Out1) -> Merge1/2
  If1/5 -> If Action Subsystem6/Action
  If Action Subsystem7/1(Out1) -> Merge1/3
  If1/3 -> If Action Subsystem7/Action
  If1/7 -> If Action Subsystem3/Action
  If Action Subsystem5/1(Out1) -> Merge1/4
  If Action Subsystem2/1(Out1) -> Merge1/10
  If1/2 -> If Action Subsystem8/Action
  If1/1 -> If Action Subsystem9/Action
  If Action Subsystem9/1(Out1) -> Merge1/1
  If Action Subsystem10/1(Out1) -> Merge1/9
  If1/9 -> If Action Subsystem10/Action

== system LUT_kidney_25/If Action Subsystem6/If Action Subsystem3/If Action Subsystem7 ==
  note: 0.7-0.79
  In1 : Inport
  Action Port : ActionPort  ActionPortLabel=elseif( u1 >= 0.695)
  From Workspace2 : FromWorkspace  VariableName=SimInputHR  Interpolate=off  OutputAfterFinalValue=Setting to zero
  If Action Subsystem1 : Subsystem  TreatAsAtomicUnit=on
  If Action Subsystem10 : Subsystem  TreatAsAtomicUnit=on
  If Action Subsystem2 : Subsystem  TreatAsAtomicUnit=on
  If Action Subsystem3 : Subsystem  TreatAsAtomicUnit=on
  If Action Subsystem4 : Subsystem  TreatAsAtomicUnit=on
  If Action Subsystem5 : Subsystem  TreatAsAtomicUnit=on
  If Action Subsystem6 : Subsystem  TreatAsAtomicUnit=on
  If Action Subsystem7 : Subsystem  TreatAsAtomicUnit=on
  If Action Subsystem8 : Subsystem  TreatAsAtomicUnit=on
  If Action Subsystem9 : Subsystem  TreatAsAtomicUnit=on
  If1 : If  IfExpression=u1 >= 0.785  ElseIfExpressions=u1 >= 0.775, u1 >= 0.765, u1 >= 0.755, u1 >= 0.745, u1 >= 0.735, u1 >= 0.725, u1 >= 0.715, u1 >= 0.705
  Merge1 : Merge  Inputs=10
  Out1 : Outport
  wires:
  If1/10 -> If Action Subsystem2/Action
  If Action Subsystem4/1(Out1) -> Merge1/6
  From Workspace2/1 -> If1/1
  If Action Subsystem6/1(Out1) -> Merge1/5
  Merge1/1 -> Out1/1
  If1/8 -> If Action Subsystem1/Action
  If Action Subsystem3/1(Out1) -> Merge1/7
  In1/1 -> If Action Subsystem1/1(In1), If Action Subsystem3/1(In1), If Action Subsystem4/1(In1), If Action Subsystem7/1(In1), If Action Subsystem8/1(In1), If Action Subsystem9/1(In1), If Action Subsystem5/1(In1), If Action Subsystem6/1(In1), If Action Subsystem10/1(In1), If Action Subsystem2/1(In1)
  If1/6 -> If Action Subsystem4/Action
  If Action Subsystem1/1(Out1) -> Merge1/8
  If1/4 -> If Action Subsystem5/Action
  If Action Subsystem8/1(Out1) -> Merge1/2
  If1/5 -> If Action Subsystem6/Action
  If Action Subsystem7/1(Out1) -> Merge1/3
  If1/3 -> If Action Subsystem7/Action
  If1/7 -> If Action Subsystem3/Action
  If Action Subsystem5/1(Out1) -> Merge1/4
  If Action Subsystem2/1(Out1) -> Merge1/10
  If1/2 -> If Action Subsystem8/Action
  If1/1 -> If Action Subsystem9/Action
  If Action Subsystem9/1(Out1) -> Merge1/1
  If1/9 -> If Action Subsystem10/Action
  If Action Subsystem10/1(Out1) -> Merge1/9

== system LUT_kidney_25/If Action Subsystem6/If Action Subsystem3/If Action Subsystem8 ==
  note: 0.8-0.89
  In1 : Inport
  Action Port : ActionPort  ActionPortLabel=elseif(u1 >= 0.795)
  From Workspace2 : FromWorkspace  VariableName=SimInputHR  Interpolate=off  OutputAfterFinalValue=Setting to zero
  If Action Subsystem1 : Subsystem  TreatAsAtomicUnit=on
  If Action Subsystem10 : Subsystem  TreatAsAtomicUnit=on
  If Action Subsystem2 : Subsystem  TreatAsAtomicUnit=on
  If Action Subsystem3 : Subsystem  TreatAsAtomicUnit=on
  If Action Subsystem4 : Subsystem  TreatAsAtomicUnit=on
  If Action Subsystem5 : Subsystem  TreatAsAtomicUnit=on
  If Action Subsystem6 : Subsystem  TreatAsAtomicUnit=on
  If Action Subsystem7 : Subsystem  TreatAsAtomicUnit=on
  If Action Subsystem8 : Subsystem  TreatAsAtomicUnit=on
  If Action Subsystem9 : Subsystem  TreatAsAtomicUnit=on
  If1 : If  IfExpression=u1 >= 0.885  ElseIfExpressions=u1 >= 0.875, u1 >= 0.865, u1 >= 0.855, u1 >= 0.845, u1 >= 0.835, u1 >= 0.825, u1 >= 0.815, u1 >= 0.805
  Merge1 : Merge  Inputs=10
  Out1 : Outport
  wires:
  If1/10 -> If Action Subsystem2/Action
  If Action Subsystem4/1(Out1) -> Merge1/6
  From Workspace2/1 -> If1/1
  If Action Subsystem6/1(Out1) -> Merge1/5
  Merge1/1 -> Out1/1
  If1/8 -> If Action Subsystem1/Action
  If Action Subsystem3/1(Out1) -> Merge1/7
  In1/1 -> If Action Subsystem1/1(In1), If Action Subsystem3/1(In1), If Action Subsystem4/1(In1), If Action Subsystem7/1(In1), If Action Subsystem8/1(In1), If Action Subsystem9/1(In1), If Action Subsystem5/1(In1), If Action Subsystem6/1(In1), If Action Subsystem10/1(In1), If Action Subsystem2/1(In1)
  If1/6 -> If Action Subsystem4/Action
  If Action Subsystem1/1(Out1) -> Merge1/8
  If1/4 -> If Action Subsystem5/Action
  If Action Subsystem8/1(Out1) -> Merge1/2
  If1/5 -> If Action Subsystem6/Action
  If Action Subsystem7/1(Out1) -> Merge1/3
  If1/3 -> If Action Subsystem7/Action
  If1/7 -> If Action Subsystem3/Action
  If Action Subsystem5/1(Out1) -> Merge1/4
  If Action Subsystem2/1(Out1) -> Merge1/10
  If1/2 -> If Action Subsystem8/Action
  If1/1 -> If Action Subsystem9/Action
  If Action Subsystem9/1(Out1) -> Merge1/1
  If1/9 -> If Action Subsystem10/Action
  If Action Subsystem10/1(Out1) -> Merge1/9

== system LUT_kidney_25/If Action Subsystem6/If Action Subsystem3/If Action Subsystem9 ==
  note: 0.9-0.99
  In2 : Inport
  Action Port : ActionPort  ActionPortLabel=if(u1 >= 0.895)
  From Workspace2 : FromWorkspace  VariableName=SimInputHR  Interpolate=off  OutputAfterFinalValue=Setting to zero
  If Action Subsystem1 : Subsystem  TreatAsAtomicUnit=on
  If Action Subsystem10 : Subsystem  TreatAsAtomicUnit=on
  If Action Subsystem2 : Subsystem  TreatAsAtomicUnit=on
  If Action Subsystem3 : Subsystem  TreatAsAtomicUnit=on
  If Action Subsystem4 : Subsystem  TreatAsAtomicUnit=on
  If Action Subsystem5 : Subsystem  TreatAsAtomicUnit=on
  If Action Subsystem6 : Subsystem  TreatAsAtomicUnit=on
  If Action Subsystem7 : Subsystem  TreatAsAtomicUnit=on
  If Action Subsystem8 : Subsystem  TreatAsAtomicUnit=on
  If Action Subsystem9 : Subsystem  TreatAsAtomicUnit=on
  If1 : If  IfExpression=u1 >= 0.985  ElseIfExpressions=u1 >= 0.975, u1 >= 0.965, u1 >= 0.955, u1 >= 0.945, u1 >= 0.935, u1 >= 0.925, u1 >= 0.915, u1 >= 0.905
  Merge1 : Merge  Inputs=10
  Out2 : Outport
  wires:
  If1/10 -> If Action Subsystem2/Action
  If Action Subsystem4/1(Out1) -> Merge1/6
  From Workspace2/1 -> If1/1
  If Action Subsystem6/1(Out1) -> Merge1/5
  Merge1/1 -> Out2/1
  If1/8 -> If Action Subsystem1/Action
  If Action Subsystem3/1(Out1) -> Merge1/7
  In2/1 -> If Action Subsystem10/1(In1), If Action Subsystem1/1(In1), If Action Subsystem3/1(In1), If Action Subsystem4/1(In1), If Action Subsystem7/1(In1), If Action Subsystem8/1(In1), If Action Subsystem9/1(In1), If Action Subsystem5/1(In1), If Action Subsystem6/1(In1), If Action Subsystem2/1(In1)
  If1/6 -> If Action Subsystem4/Action
  If Action Subsystem1/1(Out1) -> Merge1/8
  If1/4 -> If Action Subsystem5/Action
  If Action Subsystem8/1(Out1) -> Merge1/2
  If1/5 -> If Action Subsystem6/Action
  If Action Subsystem7/1(Out1) -> Merge1/3
  If1/3 -> If Action Subsystem7/Action
  If1/7 -> If Action Subsystem3/Action
  If Action Subsystem5/1(Out1) -> Merge1/4
  If Action Subsystem2/1(Out1) -> Merge1/10
  If1/2 -> If Action Subsystem8/Action
  If1/1 -> If Action Subsystem9/Action
  If Action Subsystem9/1(Out1) -> Merge1/1
  If1/9 -> If Action Subsystem10/Action
  If Action Subsystem10/1(Out1) -> Merge1/9

== system LUT_kidney_25/If Action Subsystem6/If Action Subsystem1/If Action Subsystem5/If Action Subsystem1 ==
  In1 : Inport
  Action Port : ActionPort  ActionPortLabel=elseif( u1 >= 1.115)
  LUT 1.12RR : Lookup_n-D  NumberOfTableDimensions=1  BreakpointsForDimension1=[433.4935;534.0163;632.1664;730.6368;829.0669;927.4533;1025.808;1124.139;1222.454;1320.758;1419.053;1517.342;1615.626;1713.906;1812.184;1910.459;2008.731]  Table=[400;500;600;700;800;900;1000;1100;1200;1300;1400;1500;1600;1700;1800;1900;2000]  InternalRulePriority=Speed  RndMeth=Simplest
  Out1 : Outport
  wires:
  In1/1 -> LUT 1.12RR/1
  LUT 1.12RR/1 -> Out1/1

== system LUT_kidney_25/If Action Subsystem6/If Action Subsystem1/If Action Subsystem5/If Action Subsystem10 ==
  In1 : Inport
  Action Port : ActionPort  ActionPortLabel=elseif( u1 >= 1.105)
  LUT 1.11RR : Lookup_n-D  NumberOfTableDimensions=1  BreakpointsForDimension1=[433.6133;534.1951;632.4145;730.9627;829.4755;927.948;1026.391;1124.812;1223.218;1321.613;1420.001;1518.383;1616.76;1715.134;1813.506;1911.875;2010.241]  Table=[400;500;600;700;800;900;1000;1100;1200;1300;1400;1500;1600;1700;1800;1900;2000]  InternalRulePriority=Speed  RndMeth=Simplest
  Out1 : Outport
  wires:
  In1/1 -> LUT 1.11RR/1
  LUT 1.11RR/1 -> Out1/1

== system LUT_kidney_25/If Action Subsystem6/If Action Subsystem1/If Action Subsystem5/If Action Subsystem2 ==
  In1 : Inport
  Action Port : ActionPort  ActionPortLabel=else
  LUT 1.10RR : Lookup_n-D  NumberOfTableDimensions=1  BreakpointsForDimension1=[433.7354;534.3781;632.6688;731.2967;829.8942;928.4546;1026.987;1125.5;1223.999;1322.488;1420.97;1519.447;1617.919;1716.389;1814.857;1913.322;2011.784]  Table=[400;500;600;700;800;900;1000;1100;1200;1300;1400;1500;1600;1700;1800;1900;2000]  InternalRulePriority=Speed  RndMeth=Simplest
  Out1 : Outport
  wires:
  In1/1 -> LUT 1.10RR/1
  LUT 1.10RR/1 -> Out1/1

== system LUT_kidney_25/If Action Subsystem6/If Action Subsystem1/If Action Subsystem5/If Action Subsystem3 ==
  In1 : Inport
  Action Port : ActionPort  ActionPortLabel=elseif( u1 >= 1.125)
  LUT 1.13RR : Lookup_n-D  NumberOfTableDimensions=1  BreakpointsForDimension1=[433.376;533.8414;631.9241;730.3186;828.6678;926.9702;1025.238;1123.482;1221.708;1319.922;1418.126;1516.324;1614.517;1712.705;1810.89;1909.073;2007.252]  Table=[400;500;600;700;800;900;1000;1100;1200;1300;1400;1500;1600;1700;1800;1900;2000]  InternalRulePriority=Speed  RndMeth=Simplest
  Out1 : Outport
  wires:
  In1/1 -> LUT 1.13RR/1
  LUT 1.13RR/1 -> Out1/1

== system LUT_kidney_25/If Action Subsystem6/If Action Subsystem1/If Action Subsystem5/If Action Subsystem4 ==
  In1 : Inport
  Action Port : ActionPort  ActionPortLabel=elseif( u1 >= 1.135)
  LUT 1.14RR : Lookup_n-D  NumberOfTableDimensions=1  BreakpointsForDimension1=[433.2606;533.6705;631.6875;730.008;828.2782;926.4983;1024.682;1122.839;1220.978;1319.104;1417.22;1515.328;1613.431;1711.529;1809.624;1907.716;2005.805]  Table=[400;500;600;700;800;900;1000;1100;1200;1300;1400;1500;1600;1700;1800;1900;2000]  InternalRulePriority=Speed  RndMeth=Simplest
  Out1 : Outport
  wires:
  In1/1 -> LUT 1.14RR/1
  LUT 1.14RR/1 -> Out1/1

== system LUT_kidney_25/If Action Subsystem6/If Action Subsystem1/If Action Subsystem5/If Action Subsystem5 ==
  In1 : Inport
  Action Port : ActionPort  ActionPortLabel=elseif( u1 >= 1.155)
  LUT 1.16RR : Lookup_n-D  NumberOfTableDimensions=1  BreakpointsForDimension1=[433.0358;533.3398;631.2306;729.4084;827.5258;925.5865;1023.606;1121.597;1219.566;1317.521;1415.464;1513.399;1611.328;1709.251;1807.17;1905.086;2002.999]  Table=[400;500;600;700;800;900;1000;1100;1200;1300;1400;1500;1600;1700;1800;1900;2000]  InternalRulePriority=Speed  RndMeth=Simplest
  Out1 : Outport
  wires:
  In1/1 -> LUT 1.16RR/1
  LUT 1.16RR/1 -> Out1/1

== system LUT_kidney_25/If Action Subsystem6/If Action Subsystem1/If Action Subsystem5/If Action Subsystem6 ==
  In1 : Inport
  Action Port : ActionPort  ActionPortLabel=elseif( u1 >= 1.145)
  LUT 1.15RR : Lookup_n-D  NumberOfTableDimensions=1  BreakpointsForDimension1=[433.1472;533.5033;631.4564;729.7047;827.8976;926.0371;1024.138;1122.211;1220.264;1318.304;1416.332;1514.353;1612.368;1710.378;1808.384;1906.387;2004.387]  Table=[400;500;600;700;800;900;1000;1100;1200;1300;1400;1500;1600;1700;1800;1900;2000]  InternalRulePriority=Speed  RndMeth=Simplest
  Out1 : Outport
  wires:
  In1/1 -> LUT 1.15RR/1
  LUT 1.15RR/1 -> Out1/1

== system LUT_kidney_25/If Action Subsystem6/If Action Subsystem1/If Action Subsystem5/If Action Subsystem7 ==
  In1 : Inport
  Action Port : ActionPort  ActionPortLabel=elseif( u1 >= 1.165)
  LUT 1.17RR : Lookup_n-D  NumberOfTableDimensions=1  BreakpointsForDimension1=[432.9264;533.1797;631.0099;729.1189;827.1624;925.1461;1023.086;1120.996;1218.883;1316.755;1414.615;1512.465;1610.309;1708.147;1805.982;1903.812;2001.639]  Table=[400;500;600;700;800;900;1000;1100;1200;1300;1400;1500;1600;1700;1800;1900;2000]  InternalRulePriority=Speed  RndMeth=Simplest
  Out1 : Outport
  wires:
  In1/1 -> LUT 1.17RR/1
  LUT 1.17RR/1 -> Out1/1

== system LUT_kidney_25/If Action Subsystem6/If Action Subsystem1/If Action Subsystem5/If Action Subsystem8 ==
  In1 : Inport
  Action Port : ActionPort  ActionPortLabel=elseif(u1 >= 1.175)
  LUT 1.18RR : Lookup_n-D  NumberOfTableDimensions=1  BreakpointsForDimension1=[432.8188;533.023;630.7942;728.8359;826.8073;924.7155;1022.578;1120.408;1218.215;1316.005;1413.783;1511.551;1609.312;1707.067;1804.817;1902.563;2000.306]  Table=[400;500;600;700;800;900;1000;1100;1200;1300;1400;1500;1600;1700;1800;1900;2000]  InternalRulePriority=Speed  RndMeth=Simplest
  Out1 : Outport
  wires:
  In1/1 -> LUT 1.18RR/1
  LUT 1.18RR/1 -> Out1/1

== system LUT_kidney_25/If Action Subsystem6/If Action Subsystem1/If Action Subsystem5/If Action Subsystem9 ==
  In1 : Inport
  Action Port : ActionPort  ActionPortLabel=if(u1 >= 1.185)
  LUT 1.19RR : Lookup_n-D  NumberOfTableDimensions=1  BreakpointsForDimension1=[432.713;532.8696;630.5834;728.5594;826.4602;924.2944;1022.081;1119.833;1217.561;1315.271;1412.968;1510.655;1608.334;1706.008;1803.676;1901.34;1999.001]  Table=[400;500;600;700;800;900;1000;1100;1200;1300;1400;1500;1600;1700;1800;1900;2000]  InternalRulePriority=Speed  RndMeth=Simplest
  Out1 : Outport
  wires:
  In1/1 -> LUT 1.19RR/1
  LUT 1.19RR/1 -> Out1/1

== system LUT_kidney_25/If Action Subsystem6/If Action Subsystem1/If Action Subsystem6/If Action Subsystem1 ==
  In1 : Inport
  Action Port : ActionPort  ActionPortLabel=elseif( u1 >= 1.015)
  LUT 1.02RR : Lookup_n-D  NumberOfTableDimensions=1  BreakpointsForDimension1=[434.8086;536.0154;634.9534;734.2975;833.6507;932.992;1032.323;1131.646;1230.964;1330.278;1429.591;1528.903;1628.215;1727.526;1826.838;1926.148;2025.453]  Table=[400;500;600;700;800;900;1000;1100;1200;1300;1400;1500;1600;1700;1800;1900;2000]  InternalRulePriority=Speed  RndMeth=Simplest
  Out1 : Outport
  wires:
  In1/1 -> LUT 1.02RR/1
  LUT 1.02RR/1 -> Out1/1

== system LUT_kidney_25/If Action Subsystem6/If Action Subsystem1/If Action Subsystem6/If Action Subsystem10 ==
  In1 : Inport
  Action Port : ActionPort  ActionPortLabel=elseif( u1 >= 1.005)
  LUT 1.01RR : Lookup_n-D  NumberOfTableDimensions=1  BreakpointsForDimension1=[434.9567;536.2449;635.2748;734.7194;834.1779;933.6278;1033.069;1132.504;1231.935;1331.364;1430.791;1530.218;1629.645;1729.073;1828.5;1927.927;2027.347]  Table=[400;500;600;700;800;900;1000;1100;1200;1300;1400;1500;1600;1700;1800;1900;2000]  InternalRulePriority=Speed  RndMeth=Simplest
  Out1 : Outport
  wires:
  In1/1 -> LUT 1.01RR/1
  LUT 1.01RR/1 -> Out1/1

== system LUT_kidney_25/If Action Subsystem6/If Action Subsystem1/If Action Subsystem6/If Action Subsystem2 ==
  In1 : Inport
  Action Port : ActionPort  ActionPortLabel=else
  LUT 1.00RR : Lookup_n-D  NumberOfTableDimensions=1  BreakpointsForDimension1=[435.1083;536.4808;635.6053;735.1532;834.7198;934.2808;1033.835;1133.385;1232.932;1332.477;1432.021;1531.566;1631.112;1730.658;1830.205;1929.75;2029.288]  Table=[400;500;600;700;800;900;1000;1100;1200;1300;1400;1500;1600;1700;1800;1900;2000]  InternalRulePriority=Speed  RndMeth=Simplest
  Out1 : Outport
  wires:
  In1/1 -> LUT 1.00RR/1
  LUT 1.00RR/1 -> Out1/1

== system LUT_kidney_25/If Action Subsystem6/If Action Subsystem1/If Action Subsystem6/If Action Subsystem3 ==
  In1 : Inport
  Action Port : ActionPort  ActionPortLabel=elseif( u1 >= 1.025)
  LUT 1.03RR : Lookup_n-D  NumberOfTableDimensions=1  BreakpointsForDimension1=[434.664;535.7919;634.6408;733.887;833.1374;932.3729;1031.596;1130.809;1230.017;1329.22;1428.421;1527.621;1626.819;1726.017;1825.215;1924.411;2023.604]  Table=[400;500;600;700;800;900;1000;1100;1200;1300;1400;1500;1600;1700;1800;1900;2000]  InternalRulePriority=Speed  RndMeth=Simplest
  Out1 : Outport
  wires:
  In1/1 -> LUT 1.03RR/1
  LUT 1.03RR/1 -> Out1/1
